simulink model "SIMULACIONNOLINEAL"  (R2017b)
settings: Solver=ode45  StartTime=0.0  StopTime=10.0  MaxStep=0.2  RelTol=1e-3
settings Model: Creator=alfre  LastModifiedBy=alfre

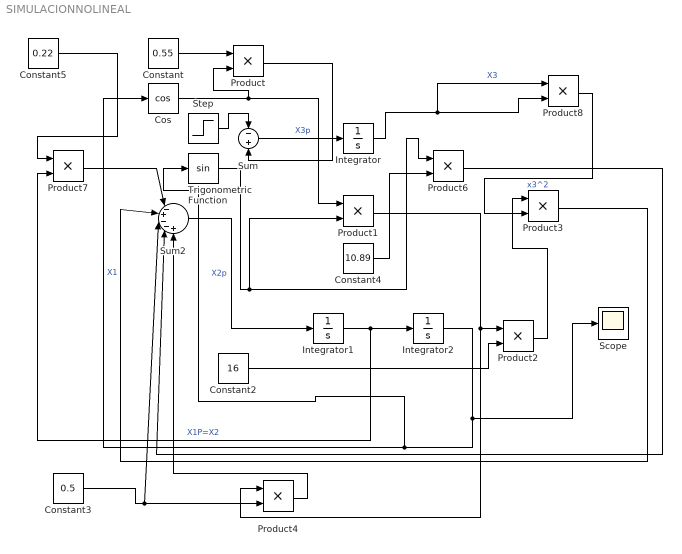
== system SIMULACIONNOLINEAL ==
  Constant : Constant  Value=0.55
  Constant2 : Constant  Value=16
  Constant3 : Constant  Value=0.5
  Constant4 : Constant  Value=10.89
  Constant5 : Constant  Value=0.22
  Cos : Trigonometry  Operator=cos
  Integrator : Integrator
  Integrator1 : Integrator
  Integrator2 : Integrator
  Product{,1..4,6..8} (8 alike) : Product
  Scope : Scope
  Step : Step  SampleTime=0
  Sum : Sum  Inputs=-+
  Sum2 : Sum  Inputs=|-+--+
  Trigonometric Function : Trigonometry
  wires:
  Sum/1 -> Integrator/1  "X3p"
  Sum2/1 -> Integrator1/1  "X2p"
  Integrator1/1 -> Product7/2, Integrator2/1  "X1P=X2"
  Integrator2/1 -> Trigonometric Function/1, Cos/1, Scope/1  "X1"
  Constant/1 -> Product/1
  Product/1 -> Sum/2
  Product8/1 -> Product3/2  "x3^2"
  Constant2/1 -> Product2/2
  Product2/1 -> Product3/1
  Product3/1 -> Sum2/2
  Constant3/1 -> Product4/2, Sum2/3
  Cos/1 -> Product1/1, Product/2
  Product4/1 -> Sum2/5
  Trigonometric Function/1 -> Product6/1, Product1/2
  Constant4/1 -> Product6/2
  Product6/1 -> Sum2/4
  Constant5/1 -> Product7/1
  Product7/1 -> Sum2/1
  Integrator/1 -> Product8/1, Product8/2  "X3"
  Product1/1 -> Product4/1, Product2/1
  Step/1 -> Sum/1
